simulink library "dspmlti2"  (Simulink 3.00)
values from neighbouring files (symbols this model uses):
  n0 = abs(a)    [dsprprim.m]
  n1 = b    [dsprprim.m]
undefined symbols (not defined in the file or in its folder): hh, hl, remez, tree
settings Model: Creator=tbryan  LastModifiedBy=sconahan

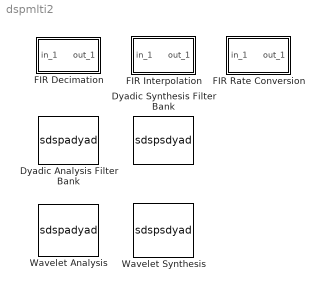
== system dspmlti2 ==
  Dyadic Analysis Filter Bank : S-Function  FunctionName=sdspadyad  Parameters=hl,hh,numLevels,tree,numChans  PortCounts=[]  SFunctionModules=''  mask(Dyadic Analysis Filter Bank){hl=fir1(12,0.4), hh=fir1(12,0.6,'high'), numLevels=2, tree=Asymmetric, frame=off, numChans=1}
      mask prompts: hl "Lowpass FIR filter coefficients:"; hh "Highpass FIR filter coefficients:"; numLevels "Number of levels:"; tree "Tree structure:"; frame "Frame-based inputs"; numChans "Number of channels:"
      mask help: Apply a sequence of FIR filters to the input signal, downsampling by two following each filtering operation. With reference to the icon on the block, a lowpass filter is applied at each descending branch and a highpass filter is applied at each non-descending branch. Normally, the lowpass and highpass filters are complementary, as in a typical wavelet-based signal decomposition.
      mask init:
      | [hl,hh,x,y,str] = dspblkadyad(hl,hh,numLevels,tree);
      | if strcmp(frame,'off'), numChans=-1; end
      mask Help: web(dspbhelp);
      mask StyleString: edit,edit,edit,popup(Asymmetric|Symmetric),checkbox,edit
      mask CallbackString: ||||dspblkadyad|
      mask Display:
      | text(0.1,0.15,str)
      | plot(x,y)
  Dyadic Synthesis Filter Bank : S-Function  FunctionName=sdspsdyad  Parameters=hl,hh,numLevels,tree,numChans  PortCounts=[]  SFunctionModules=''  mask(Dyadic Synthesis Filter Bank){hl=fir1(12,0.4), hh=fir1(12,0.6,'high'), numLevels=2, tree=Asymmetric, frame=off, numChans=1}
      mask prompts: hl "Lowpass FIR filter coefficients:"; hh "Highpass FIR filter coefficients:"; numLevels "Number of levels:"; tree "Tree structure:"; frame "Frame-based inputs"; numChans "Number of channels:"
      mask help: Apply a sequence of FIR filters to the input signals, upsampling by two following each filtering operation. With reference to the icon on the block, a lowpass filter is applied at each descending branch and a highpass filter is applied at each non-descending branch. Normally, the lowpass and highpass filters are complementary, as in a typical wavelet-based signal reconstruction.
      mask init:
      | [hl,hh,x,y,str] = dspblksdyad(hl,hh,numLevels,tree);
      | if strcmp(frame,'off'), numChans=-1; end
      mask Help: web(dspbhelp);
      mask StyleString: edit,edit,edit,popup(Asymmetric|Symmetric),checkbox,edit
      mask CallbackString: ||||dspblksdyad|
      mask Display:
      | text(0.80,0.15,str)
      | plot(x,y)
  FIR Decimation : Subsystem  mask(FIR Decimation){h=fir1(35,0.4), D=2, frame=off, numChans=1, framing=Maintain input frame size}
      mask prompts: h "FIR filter coefficients:"; D "Decimation factor:"; frame "Frame-based inputs"; numChans "Number of channels:"
      mask help: Apply an FIR filter to the input signal, then downsample by an integer factor. Implemented using an efficient polyphase FIR decimation structure.
      mask init:
      | outputBufInitCond = 0;
      | [str,numChans] = dspblkfirdn('setup1',numChans);
      | [h,framing,str] = dspblkfirdn('setup2',h,D,framing);
      mask Help: web(dspbhelp);
      mask StyleString: edit,edit,checkbox,edit,popup(Maintain input frame size|Maintain input frame rate)
      mask CallbackString: ||dspblkfirdn||
      mask Display: disp(str)
  FIR Interpolation : Subsystem  mask(FIR Interpolation){h=fir1(15,1/4), L=3, frame=off, numChans=1, framing=Maintain input frame size}
      mask prompts: h "FIR filter coefficients:"; L "Interpolation factor:"; frame "Frame-based inputs"; numChans "Number of channels:"
      mask help: Upsample input signal by an integer factor, then apply an FIR filter. Implemented using an efficient polyphase interpolation structure. The filter coefficients are scaled by the interpolation factor.
      mask init:
      | outputBufInitCond = 0;
      | [str,numChans] = dspblkupfir('setup1',numChans);
      | [h,framing,str]= dspblkupfir('setup2',h,L,framing);
      mask Help: web(dspbhelp);
      mask StyleString: edit,edit,checkbox,edit,popup(Maintain input frame size|Maintain input frame rate)
      mask CallbackString: ||dspblkupfir||
      mask Display: disp(str)
  FIR Rate Conversion : Subsystem  mask(FIR Rate Conversion){L=3, h=remez(70,[0 .28 .32 1],[1 1 0 0]), M=2, numChans=1}
      mask prompts: L "Interpolation factor:"; h "FIR filter coefficients:"; M "Decimation factor:"; numChans "Number of channels:"
      mask help: Upsample input signal by an integer factor, apply an FIR filter and downsample by another integer factor. Implemented using an efficient polyphase structure. Only frame-based processing is supported. The filter coefficients are scaled by the upsample factor. For some combinations of upsample and downsample factors there will be a delay in the output due to causality in the polyphase network.
      mask init:
      | outputBufInitCond = 0;
      | str = ['x[?]'];
      | [h,L,M,n0,n1,str]= dspblkupfirdn('setup',h,L,M);
      mask Help: web(dspbhelp);
      mask Display: disp(str)
  Wavelet Analysis : S-Function  FunctionName=sdspadyad  Parameters=hl,hh,NumLevels,tree,NumChans  PortCounts=[]  SFunctionModules=''  mask(Wavelet Analysis){Wname=Haar, OrdRec_ordDec=[1 / 1], Order=2, NumLevels=2, Frame=off, NumChans=1}
      mask prompts: Wname "Wavelet name:"; OrdRec_ordDec "Filter order [synthesis / analysis]:"; Order "Wavelet order:"; NumLevels "Number of levels:"; Frame "Frame-based inputs"; NumChans "Number of channels:"
      mask help:
      | Multilevel discrete 1-D wavelet decomposition using a specific wavelet.
      |
      | The Wavelet Toolbox must be installed to use this block.
      mask init:
      | [x,y,str] = dspblkwavedec('icon');
      | [hl, hh, tree] = dspblkwavedec('init');
      | if strcmp(Frame,'off'), NumChans=-1; end
      mask Help: web(dspbhelp);
      mask StyleString: popup(Haar|Daubechies|Symlets|Coiflets|Biorthogonal|Reverse Biorthogonal|Discrete Meyer),popup([1 / 1]|[1 / 3]|[1 / 5]|[2 / 2]|[2 / 4]|[2 / 6]|[2 / 8]|[3 / 1]|[3 / 3]|[3 / 5]|[3 / 7]|[3 / 9]|[4 / 4]|[5 / 5]|[6 / 8]),edit,edit,checkbox,edit
      mask CallbackString: dspblkwavedec||||dspblkwavedec|
      mask Display:
      | text(0.08,0.1,str)
      | plot(x,y)
  Wavelet Synthesis : S-Function  FunctionName=sdspsdyad  Parameters=hl,hh,NumLevels,tree,NumChans  PortCounts=[]  SFunctionModules=''  mask(Wavelet Synthesis){Wname=Haar, OrdRec_ordDec=[1 / 1], Order=2, NumLevels=2, Frame=off, NumChans=1}
      mask prompts: Wname "Wavelet name:"; OrdRec_ordDec "Filter order [synthesis, analysis]:"; Order "Wavelet order:"; NumLevels "Number of levels:"; Frame "Frame-based inputs"; NumChans "Number of channels:"
      mask help:
      | Multilevel discrete 1-D wavelet reconstruction using a specific wavelet.
      |
      | The Wavelet Toolbox must be installed to use this block.
      mask init:
      | [x,y,str] = dspblkwaverec('icon');
      | [hl, hh, tree] = dspblkwaverec('init');
      | if strcmp(Frame,'off'), NumChans=-1; end
      mask Help: web(dspbhelp);
      mask StyleString: popup(Haar|Daubechies|Symlets|Coiflets|Biorthogonal|Reverse Biorthogonal|Discrete Meyer),popup([1 / 1]|[1 / 3]|[1 / 5]|[2 / 2]|[2 / 4]|[2 / 6]|[2 / 8]|[3 / 1]|[3 / 3]|[3 / 5]|[3 / 7]|[3 / 9]|[4 / 4]|[5 / 5]|[6 / 8]),edit,edit,checkbox,edit
      mask CallbackString: dspblkwaverec||||dspblkwaverec|
      mask Display:
      | text(0.37,0.15,str)
      | plot(x,y)

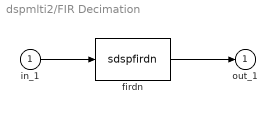
== system dspmlti2/FIR Decimation ==
  in_1 : Inport  Port=1  PortWidth=-1  SampleTime=-1  DataType=auto
      settings: SignalType=auto
  firdn : S-Function  FunctionName=sdspfirdn  Parameters=h,D,numChans,framing,outputBufInitCond  PortCounts=[]  SFunctionModules=''
  out_1 : Outport  Port=1  InitialOutput=0
  wires:
  in_1/1 -> firdn/1
  firdn/1 -> out_1/1

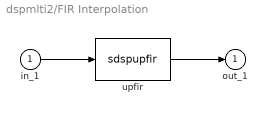
== system dspmlti2/FIR Interpolation ==
  in_1 : Inport  Port=1  PortWidth=-1  SampleTime=-1  DataType=auto
      settings: SignalType=auto
  upfir : S-Function  FunctionName=sdspupfir  Parameters=h,L,numChans,framing,outputBufInitCond  PortCounts=[]  SFunctionModules=''
  out_1 : Outport  Port=1  InitialOutput=0
  wires:
  upfir/1 -> out_1/1
  in_1/1 -> upfir/1

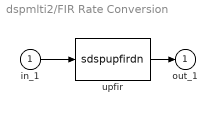
== system dspmlti2/FIR Rate Conversion ==
  in_1 : Inport  Port=1  PortWidth=-1  SampleTime=-1  DataType=auto
      settings: SignalType=auto
  upfir : S-Function  FunctionName=sdspupfirdn  Parameters=h,L,M,n0,n1,numChans,outputBufInitCond  PortCounts=[]  SFunctionModules=''
  out_1 : Outport  Port=1  InitialOutput=0
  wires:
  in_1/1 -> upfir/1
  upfir/1 -> out_1/1
